simulink model "part2"  (R2017a)
settings: Solver=VariableStepAuto  StartTime=0.0  StopTime=10.0  RelTol=1e-3
libraries: simulink x1
settings Model: Creator=user  LastModifiedBy=user

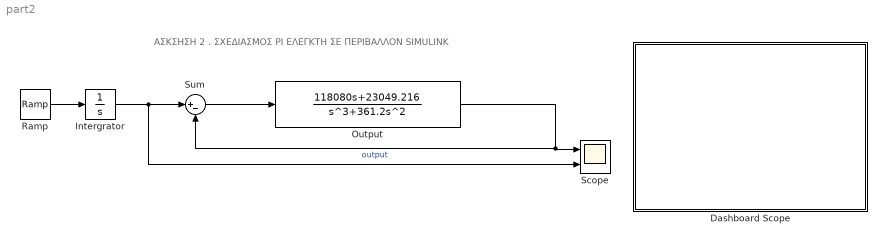
== system part2 ==
  note: ΑΣΚΣΗΣΗ 2 . ΣΧΕΔΙΑΣΜΟΣ PI ΕΛΕΓΚΤΗ ΣΕ ΠΕΡΙΒΑΛΛΟΝ SIMULINK
  Dashboard Scope : Subsystem  DialogController=hmiCreateDDGDialog  IsWebBlock=on  mask(MWDashboardBlock){webBlockId=62ba45a5-1484-4eb0-891b-543936204a4d, webBlockType=sdiscope, ShowInitialText=on, HMISrcModelName=part2}
      mask prompts: webBlockId "WebBlock Id"; webBlockType "WebBlock Type"; HMISrcModelName "Source Model"
      mask help: SimulinkHMI:dialogs:HMIScopeDialogDesc
      mask Help: helpview([docroot '/mapfiles/simulink.map'], 'hmi_scope')
      mask Display:
      | if strcmp(get_param(bdroot(gcb),'BlockDiagramType'), 'library')
      |     image([(matlabroot) '/toolbox/simulink/hmi/icons/DashboardScope.png']);
      | end
  "Intergrator " : Integrator
  Output : TransferFcn  Numerator=[118080 23049.216]  Denominator=[1 361.2 0 0]
  Ramp : simulink/Sources/Ramp  slope=1  start=0  X0=0
  Scope : Scope  NumInputPorts=2
  Sum : Sum  Inputs=|+-
  wires:
  Output/1 -> Sum/2, Scope/1  "output"
  Sum/1 -> Output/1
  Ramp/1 -> "Intergrator "/1
  "Intergrator "/1 -> Scope/2, Sum/1

== system part2/Dashboard Scope ==
